simulink model "PowerLimiting_Current_Feedback"  (R2024a)
settings: Solver=VariableStepAuto  StartTime=0.0  StopTime=97.91  RelTol=1e-3
undefined symbols (not defined in the file or in its folder): Ion, Lithium
libraries: simulink x2, spsBatteryLib x1, spsControlledCurrentSourceLib x1, slpidlib x1, spsVoltageMeasurementLib x1, spspowerguiLib x1
settings Model: Creator=ezeki  LastModifiedBy=ezeki
settings DataIOCC: ExternalInput=[throttle]

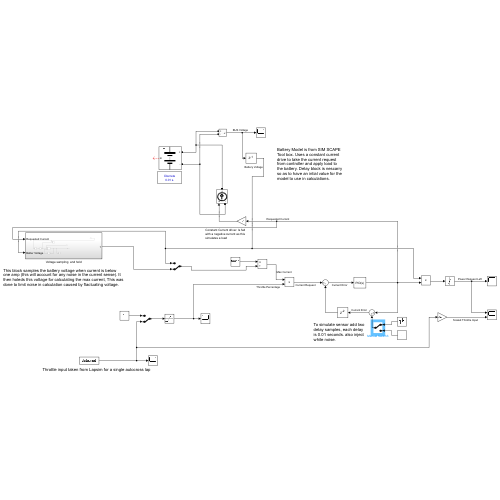
[thumbnail: Simulink's stored preview of the top-level diagram]
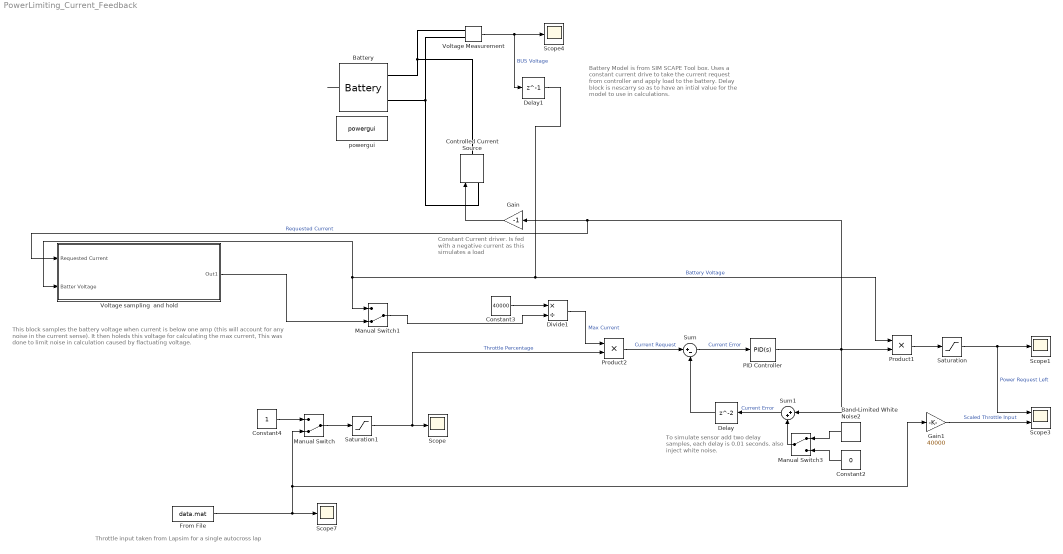
== system PowerLimiting_Current_Feedback ==
  note: Throttle input taken from Lapsim for a single autocross lap
  note: Constant Current driver. Is fed with a negative current as this simulates a load
  note: Battery Model is from SIM SCAPE Tool box. Uses a constant current drive to take the current request from controller and apply load to the battery. Delay block is nescarry so as to have an intial value for the model to use in calculations.
  note: This block samples the battery voltage when current is below one amp (this will account for any noise in the current sense). It then holeds this voltage for calculating the max current, This was done to limit noise in calculation caused by flactuating voltage.
  note: To simulate sensor add two delay samples, each delay is 0.01 seconds. also inject white noise.
  Band-Limited White Noise2 : simulink/Sources/Band-Limited White Noise  Cov=[0.1]  Ts=0.1  seed=[23341]
  Battery : spsBatteryLib/Battery  BatType=Lithium-Ion  ShowTempParam=off  ThermalPreset=no  ShowAgeParam=off  NomV=532.8  NomQ=1152  SOC=98.5  Batt_Tr=5  PresetModel=on  MaxQ=1152  MinV=399.6  FullV=620.1723  Dis_rate=500.8696  R=0.004625  Normal_OP=1041.8087  expZone="[575.6296      56.59826]"  current=[6.5 13 32.5]  Units=Time  Tci=20  NomT=20  T2=-30  MaxQ2=4.8  FullV2=7.1  Normal_OP2=5.655  expZone2="[6.58           1]"  Rca=0.6  ti=2000  Dp=0  Neq0=0  Tsim=1e6  Ta1=25  Qeol=5.4*0.9  Reol=0.013333*1.2  Char_age=[2.3478, 3]  Dis_age=[2.3478, 10]  N1=1500  N2=10500  N3=1000  N4=1400  Ta2=45  N5=950
  Constant2 : Constant  Value=0
  Constant3 : Constant  Value=40000
  Constant4 : Constant
  Controlled Current Source : spsControlledCurrentSourceLib/Controlled Current Source  Initialize=on  Source_Type=AC  Amplitude=0  Phase=0  Frequency=0  Measurements=None
  Delay : Delay
  Delay1 : Delay  DelayLength=1  InitialCondition=600
  Divide1 : Product  Inputs=*/
  From File : FromFile  FileName=data.mat  SampleTime=0
  Gain : Gain  Gain=-1
  Gain1 : Gain  Gain=40000
  Manual Switch : ManualSwitch  CurrentSetting=0
  Manual Switch1 : ManualSwitch  CurrentSetting=0
  Manual Switch3 : ManualSwitch
  PID Controller : slpidlib/PID Controller  Controller=PID  Form=Parallel  TimeDomain=Continuous-time  UseExternalTs=off  SampleTime=-1  IntegratorMethod=Forward Euler  FilterMethod=Forward Euler  ControllerParametersSource=internal  P=0  I=18.7598026660823  UseKiTs=off  D=0  UseExternalDerivativeSource=off  N=100  UseFilter=on  TunerSelectOption=Transfer Function Based (PID Tuner App)  InitialConditionSource=internal  InitialConditionForIntegrator=0  InitialConditionForFilter=0  DifferentiatorICPrevScaledInput=0  ExternalReset=none  TrackingMode=off  Kt=1  LimitOutput=off  SatLimitsSource=internal  UpperSaturationLimit=inf  LowerSaturationLimit=-inf  LinearizeAsGain=on  AntiWindupMode=none  Kb=1  LimitIntegrator=off  UpperIntegratorSaturationLimit=inf  LowerIntegratorSaturationLimit=-inf  POutMin=[]  POutMax=[]  IOutMin=[]  IOutMax=[]  DOutMin=[]  DOutMax=[]  NOutMin=[]  NOutMax=[]  SumOutMin=[]  SumOutMax=[]  SaturationOutMin=[]  SaturationOutMax=[]  PParamMin=[]  PParamMax=[]  IParamMin=[]  IParamMax=[]  DParamMin=[]  DParamMax=[]  NParamMin=[]  NParamMax=[]  KbParamMin=[]  KbParamMax=[]  KtParamMin=[]  KtParamMax=[]  KbOutMin=[]  KbOutMax=[]  KtOutMin=[]  KtOutMax=[]  IntegratorOutMin=[]  IntegratorOutMax=[]  FilterOutMin=[]  FilterOutMax=[]  SumI1OutMin=[]  SumI1OutMax=[]  SumI2OutMin=[]  SumI2OutMax=[]  SumI3OutMin=[]  SumI3OutMax=[]  SumI4OutMin=[]  SumI4OutMax=[]  SumDOutMin=[]  SumDOutMax=[]  DifferentiatorOutMin=[]  DifferentiatorOutMax=[]  FilterDiffOutCoefMin=[]  FilterDiffOutCoefMax=[]  ReciprocalOutMin=[]  ReciprocalOutMax=[]  SumDenOutMin=[]  SumDenOutMax=[]  SumNumOutMin=[]  SumNumOutMax=[]  DivideOutMin=[]  DivideOutMax=[]  UdiffTsProdOutMin=[]  UdiffTsProdOutMax=[]  NTsProdOutMin=[]  NTsProdOutMax=[]  UintegralTsProdOutMin=[]  UintegralTsProdOutMax=[]  UngainTsProdOutMin=[]  UngainTsProdOutMax=[]  ClampingZeroOutDataTypeStr=Inherit: Inherit via back propagation  ClampingZeroOutMin=[]  ClampingZeroOutMax=[]  FilterDenConstantOutDataTypeStr=Inherit: Inherit via back propagation  FilterDenConstantOutMin=[]  FilterDenConstantOutMax=[]  PCopyOutDataTypeStr=Inherit: Inherit via back propagation  PCopyOutMin=[]  PCopyOutMax=[]  NCopyOutDataTypeStr=Inherit: Inherit via back propagation  NCopyOutMin=[]  NCopyOutMax=[]  IntegratorContinuousStateAttributes=''  IntegratorStateMustResolveToSignalObject=off  IntegratorRTWStateStorageClass=Auto  FilterContinuousStateAttributes=''  FilterStateMustResolveToSignalObject=off  FilterRTWStateStorageClass=Auto  ParallelPVariant=InternalParameters  IdealPVariant=Disabled  IVariant=InternalParameters  DVariant=InternalParameters  IntegratorVariant=Continuous  SatVariant=Disabled  AWVariant=Passthrough  PCopyVariant=Disabled  TRVariant=Disabled  FdbkBlocksVariant=Forward  IdealPFdbkVariant=Disabled  SatFdbkVariant=Disabled  DerivativeFilterVariant=ContFilter  NVariant=InternalParameters  NCopyVariant=Disabled  FilterICVariant=InternalICsFilter  IntegratorICVariant=InternalICs  ExternalResetVariant=Disabled  TRSumVariant=Passthrough  SumFdbkVariant=Disabled  SumVariant=Sum_PID  TsampFilterVariant=InternalTs  TsampNgainVariant=Passthrough  TsampIntegralVariant=Disabled_SignalSpec  ExternalSaturationOutDataTypeStr=Inherit: Same as second input  DerivativeSourceVariant=ErrorSignal
  Product1 : Product
  Product2 : Product
  Saturation : Saturate  UpperLimit=inf  LowerLimit=0
  Saturation1 : Saturate  UpperLimit=inf  LowerLimit=0
  Scope{,1,4,7} (4 alike) : Scope
  Scope3 : Scope  NumInputPorts=2
  Sum : Sum  Inputs=|+-
  Sum1 : Sum  Inputs=|++
  Voltage Measurement : spsVoltageMeasurementLib/Voltage Measurement  PhasorSimulation=off  OutputType=Complex  PSBequivalent=0
  Voltage sampling  and hold : Subsystem
  powergui : spspowerguiLib/powergui  Priority=1  SimulationMode=Discrete  SampleTime=0.01  frequency=60  Iterations=50  frequencyindice=0  Pbase=100e6  ErrMax=1e-4  UnitsV=kV  UnitsW=MW  buscounter=0  FunctionMessages=off  echomessages=off  EnableUseOfTLC=off  CurrentSourceSwitches=off  DisableSnubberDevices=off  DisableRonSwitches=off  DisableVfSwitches=off  DisplayEquations=off  AutomaticDiscreteSolvers=off  SolverType=Tustin/Backward Euler (TBE)  Interpol=off  ExternalGateDelay=off  methode=off  Ts=100  x0status=blocks  SPID=on  SwTol=0  HookPort=off  NonlinearTolerance=1e-4  nMaxIteration=100  ContinueOnMaxIteration=off  RestoreLinks=warning  ResistiveCurrentMeasurement=off  Frange=[0:2:500]  Ylog=off  Xlog=on  ShowGrid=off  save=off  variable=ZData  structure=0  ZoomFFT=off  StartTime=0.0  cycles=1  DisplayStyle=1  fundamental=60  FreqAxis=off  MaxFrequency=1000  frequencyindicesteady=1  RmsSteady=1  display=off
  wires:
  Sum/1 -> PID Controller/1  "Current Error"
  Saturation1/1 -> Scope/1, Product2/2  "Throttle Percentage"
  Divide1/1 -> Product2/1  "Max Current"
  Constant4/1 -> Manual Switch/1
  Manual Switch/1 -> Saturation1/1
  Constant3/1 -> Divide1/1
  Gain/1 -> Controlled Current Source/1
  Voltage Measurement/1 -> Delay1/1, Scope4/1  "BUS Voltage"
  Delay1/1 -> Product1/1, Manual Switch1/1, Voltage sampling  and hold/2(Batter Voltage)  "Battery Voltage"
  Battery/1 -> ?
  Delay/1 -> Sum/2
  Product2/1 -> Sum/1  "Current Request"
  Sum1/1 -> Delay/1  "Current Error"
  PID Controller/1 -> Product1/2, Sum1/1, Voltage sampling  and hold/1(Requested Current), Gain/1  "Requested Current"
  Product1/1 -> Saturation/1
  From File/1 -> Scope7/1, Gain1/1, Manual Switch/2
  Manual Switch1/1 -> Divide1/2
  Constant2/1 -> Manual Switch3/2
  Manual Switch3/1 -> Sum1/2
  Band-Limited White Noise2/1 -> Manual Switch3/1
  Voltage sampling  and hold/1(Out1) -> Manual Switch1/2
  Saturation/1 -> Scope3/1, Scope1/1  "Power Request Left"
  Gain1/1 -> Scope3/2  "Scaled Throttle Input"
  connections:
  Battery/LConn1 -- Voltage Measurement/LConn1 -- Controlled Current Source/RConn1
  Controlled Current Source/LConn1 -- Battery/LConn2 -- Voltage Measurement/LConn2

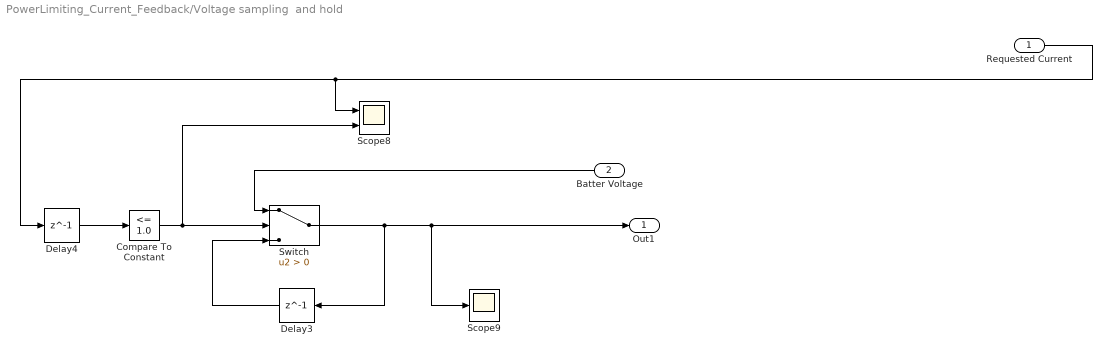
== system PowerLimiting_Current_Feedback/Voltage sampling  and hold ==
  Requested Current : Inport
  Batter Voltage : Inport  Port=2
  Compare To Constant : simulink/Logic and Bit Operations/Compare To Constant  relop=<=  const=1.0  OutDataTypeStr=boolean
  Delay3 : Delay  DelayLength=1  InitialCondition=500
  Delay4 : Delay  DelayLength=1  InitialCondition=0
  Scope8 : Scope  NumInputPorts=2
  Scope9 : Scope
  Switch : Switch  Criteria=u2 > Threshold  SaturateOnIntegerOverflow=off  InputSameDT=off
  Out1 : Outport
  wires:
  Compare To Constant/1 -> Scope8/2, Switch/2
  Requested Current/1 -> Delay4/1, Scope8/1
  Delay3/1 -> Switch/3
  Switch/1 -> Delay3/1, Out1/1, Scope9/1
  Batter Voltage/1 -> Switch/1
  Delay4/1 -> Compare To Constant/1
